simulink model "needle3"  (R2015a)
settings: Solver=ode45  StartTime=0.0  StopTime=10  FixedStep=0.01  RelTol=1e-3
settings Model: Creator=LAB425  LastModifiedBy=LAB425

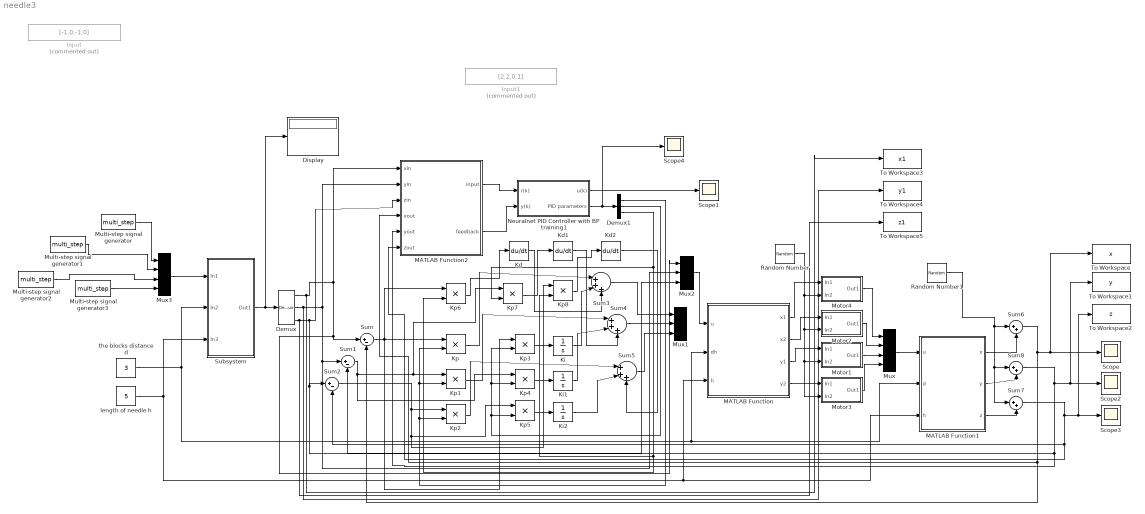
== system needle3 ==
  Demux : Demux  Outputs=3
  Demux1 : Demux  Outputs=3
  Display : Display
  Input : Constant  Commented=on  Value=[-1,0,-1,0]
  Input1 : Constant  Commented=on  Value=[2,2,0,1]
  Kd : Derivative
  Kd1 : Derivative
  Kd2 : Derivative
  "Ki " : Integrator
  Ki1 : Integrator
  Ki2 : Integrator
  Kp{,1..8} (9 alike) : Product
  MATLAB Function : MATLAB Function  TreatAsAtomicUnit=on
  MATLAB Function1 : MATLAB Function  TreatAsAtomicUnit=on
  MATLAB Function2 : MATLAB Function  TreatAsAtomicUnit=on
  Motor1 : Subsystem
  Motor2 : Subsystem
  Motor3 : Subsystem
  Motor4 : Subsystem
  Multi-step signal generator : S-Function  FunctionName=multi_step  Parameters=tTime,yStep  mask{tTime=[0,5], yStep=[-2,-1]}
      mask prompts: tTime "Time instances"; yStep "Step Values"
      mask init:
      | xx=repmat(tTime,2,1); yy=repmat(yStep,2,1);
      | xx=[xx(:)' 2*tTime(end)-tTime(end-1)];
      | yy=[0, yy(:)'];
      mask Display: plot(xx,yy)
  Multi-step signal generator1 : S-Function  FunctionName=multi_step  Parameters=tTime,yStep  mask{tTime=[0,5], yStep=[0.5,0]}
      mask prompts: tTime "Time instances"; yStep "Step Values"
      mask init:
      | xx=repmat(tTime,2,1); yy=repmat(yStep,2,1);
      | xx=[xx(:)' 2*tTime(end)-tTime(end-1)];
      | yy=[0, yy(:)'];
      mask Display: plot(xx,yy)
  Multi-step signal generator2 : S-Function  FunctionName=multi_step  Parameters=tTime,yStep  mask{tTime=[0,5], yStep=[-2,0]}
      mask prompts: tTime "Time instances"; yStep "Step Values"
      mask init:
      | xx=repmat(tTime,2,1); yy=repmat(yStep,2,1);
      | xx=[xx(:)' 2*tTime(end)-tTime(end-1)];
      | yy=[0, yy(:)'];
      mask Display: plot(xx,yy)
  Multi-step signal generator3 : S-Function  FunctionName=multi_step  Parameters=tTime,yStep  mask{tTime=[0,5], yStep=[1,0]}
      mask prompts: tTime "Time instances"; yStep "Step Values"
      mask init:
      | xx=repmat(tTime,2,1); yy=repmat(yStep,2,1);
      | xx=[xx(:)' 2*tTime(end)-tTime(end-1)];
      | yy=[0, yy(:)'];
      mask Display: plot(xx,yy)
  Mux : Mux
  Mux1 : Mux  Inputs=3
  Mux2 : Mux  Inputs=3
  Mux3 : Mux
  Neuralnet PID Controller with BP training1 : Subsystem  mask{xite=0.3, alfa=0.04, n_hidden=5, U_m=10, T=0.001, kFunc1=log-sigmoid, kFunc2=log-simoid}
      mask prompts: xite "The value of  xite"; alfa "The value of alfa"; n_hidden "number of hidden layer nodes"; U_m "Actuator Limit U_m"; T "Sampling period"; kFunc1 "Hidden Layer Trans Function"; kFunc2 "Output layer trans function"
      mask TypeOptions kFunc1: sigmoid | log-sigmoid
      mask TypeOptions kFunc2: sigmoid | log-simoid
      mask Display: disp('BP PID Controller')
  Random Number : RandomNumber  Variance=0.0005  SampleTime=0.01
  Random Number1 : RandomNumber  Variance=0.0005  Seed=1  SampleTime=0.01
  Scope{,1..4} (5 alike) : Scope
      Scope2 settings: SaveName=ScopeData2
      Scope3 settings: SaveName=ScopeData3
      Scope4 settings: SaveName=ScopeData4
  Subsystem : Subsystem
  Sum : Sum  Inputs=|+-
  Sum1 : Sum  Inputs=|+-
  Sum2 : Sum  Inputs=|+-
  Sum3 : Sum  Inputs=|+++
  Sum4 : Sum  Inputs=|+++
  Sum5 : Sum  Inputs=|+++
  Sum6 : Sum  Inputs=|++
  Sum7 : Sum  Inputs=|++
  Sum8 : Sum  Inputs=|++
  To Workspace : ToWorkspace  VariableName=x  SaveFormat=Timeseries  SampleTime=-1
  To Workspace1 : ToWorkspace  VariableName=y  SaveFormat=Timeseries  SampleTime=-1
  To Workspace2 : ToWorkspace  VariableName=z  SaveFormat=Timeseries  SampleTime=-1
  To Workspace3 : ToWorkspace  VariableName=x1  SaveFormat=Timeseries  SampleTime=-1
  To Workspace4 : ToWorkspace  VariableName=y1  SaveFormat=Timeseries  SampleTime=-1
  To Workspace5 : ToWorkspace  VariableName=z1  SaveFormat=Timeseries  SampleTime=-1
  length of needle h : Constant  Value=5
  the blocks distance d : Constant  Value=3
  wires:
  length of needle h/1 -> MATLAB Function/3(h), MATLAB Function1/3(h), Subsystem/3(In3)
  the blocks distance d/1 -> Subsystem/2(In2), MATLAB Function/2(dh), MATLAB Function1/2(d)
  Mux/1 -> MATLAB Function1/1(u)
  Motor3/1(Out1) -> Mux/4
  Mux3/1 -> Subsystem/1(In1)
  Subsystem/1(Out1) -> Display/1, Demux/1
  Random Number/1 -> Motor4/2(In2), Motor2/2(In2), Motor1/2(In2), Motor3/2(In2)
  MATLAB Function/4(y2) -> Motor3/1(In1)
  MATLAB Function/1(x1) -> Motor4/1(In1)
  MATLAB Function/2(x2) -> Motor2/1(In1)
  MATLAB Function/3(y1) -> Motor1/1(In1)
  Motor4/1(Out1) -> Mux/1
  Motor2/1(Out1) -> Mux/2
  Motor1/1(Out1) -> Mux/3
  Demux/2 -> To Workspace4/1, MATLAB Function2/2(yin), Mux2/2, Sum1/1
  Demux/3 -> To Workspace5/1, Mux2/3, Sum2/1, MATLAB Function2/3(zin)
  MATLAB Function2/2(feedback) -> Neuralnet PID Controller with BP training1/2(y(k))
  Neuralnet PID Controller with BP training1/2(PID parameters) -> Scope4/1, Demux1/1
  Sum/1 -> Kp6/1, Kp3/1, Kp/1
  Demux1/1 -> Kp/2, Kp1/2, Kp2/2
  Sum1/1 -> Kp7/1, Kp1/1, Kp4/1
  Sum2/1 -> Kp8/1, Kp5/1, Kp2/1
  Demux1/2 -> Kp3/2, Kp4/2, Kp5/2
  Kp3/1 -> "Ki "/1
  "Ki "/1 -> Sum3/2
  Kp/1 -> Sum3/1
  Kp4/1 -> Ki1/1
  Kp5/1 -> Ki2/1
  Kp1/1 -> Sum4/1
  Ki1/1 -> Sum4/2
  Sum3/1 -> Mux1/1
  Sum4/1 -> Mux1/2
  Sum5/1 -> Mux1/3
  Ki2/1 -> Sum5/2
  Kp2/1 -> Sum5/1
  Demux1/3 -> Kp8/2, Kp6/2, Kp7/2
  Kp6/1 -> Kd/1
  Kd/1 -> Sum3/3
  Kp7/1 -> Kd1/1
  Kd1/1 -> Sum4/3
  Kp8/1 -> Kd2/1
  Kd2/1 -> Sum5/3
  MATLAB Function2/1(input) -> Neuralnet PID Controller with BP training1/1(r(k))
  Demux/1 -> To Workspace3/1, MATLAB Function2/1(xin), Sum/1, Mux2/1
  Mux2/1 -> MATLAB Function/1(u)
  Neuralnet PID Controller with BP training1/1(u(k)) -> Scope1/1
  Random Number1/1 -> Sum7/1, Sum8/1, Sum6/1
  MATLAB Function1/1(x) -> Sum6/2
  Sum8/1 -> MATLAB Function2/5(yout), Sum1/2, To Workspace1/1, Scope2/1
  Sum7/1 -> MATLAB Function2/6(zout), Sum2/2, Scope3/1, To Workspace2/1
  MATLAB Function1/2(y) -> Sum8/2
  MATLAB Function1/3(z) -> Sum7/2
  Sum6/1 -> MATLAB Function2/4(xout), Sum/2, To Workspace/1, Scope/1
  Multi-step signal generator/1 -> Mux3/1
  Multi-step signal generator1/1 -> Mux3/2
  Multi-step signal generator2/1 -> Mux3/3
  Multi-step signal generator3/1 -> Mux3/4

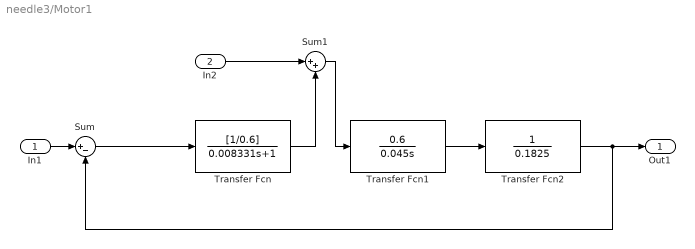
== system needle3/Motor1 ==
  In1 : Inport
  In2 : Inport  Port=2
  Sum : Sum  Inputs=|+-
  Sum1 : Sum  Inputs=|++
  Transfer Fcn : TransferFcn  Numerator=[1/0.6]  Denominator=[0.008331 1]
  Transfer Fcn1 : TransferFcn  Numerator=[0.6]  Denominator=[0.045 0]
  Transfer Fcn2 : TransferFcn  Denominator=[0.1825]
  Out1 : Outport
  wires:
  Transfer Fcn2/1 -> Sum/2, Out1/1
  Transfer Fcn1/1 -> Transfer Fcn2/1
  Sum1/1 -> Transfer Fcn1/1
  In2/1 -> Sum1/1
  Transfer Fcn/1 -> Sum1/2
  Sum/1 -> Transfer Fcn/1
  In1/1 -> Sum/1

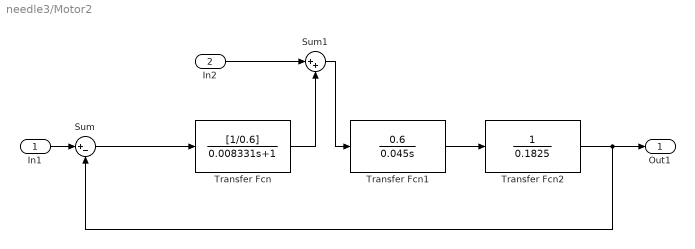
== system needle3/Motor2 ==
  In1 : Inport
  In2 : Inport  Port=2
  Sum : Sum  Inputs=|+-
  Sum1 : Sum  Inputs=|++
  Transfer Fcn : TransferFcn  Numerator=[1/0.6]  Denominator=[0.008331 1]
  Transfer Fcn1 : TransferFcn  Numerator=[0.6]  Denominator=[0.045 0]
  Transfer Fcn2 : TransferFcn  Denominator=[0.1825]
  Out1 : Outport
  wires:
  Transfer Fcn2/1 -> Sum/2, Out1/1
  Transfer Fcn1/1 -> Transfer Fcn2/1
  Sum1/1 -> Transfer Fcn1/1
  In2/1 -> Sum1/1
  Transfer Fcn/1 -> Sum1/2
  Sum/1 -> Transfer Fcn/1
  In1/1 -> Sum/1

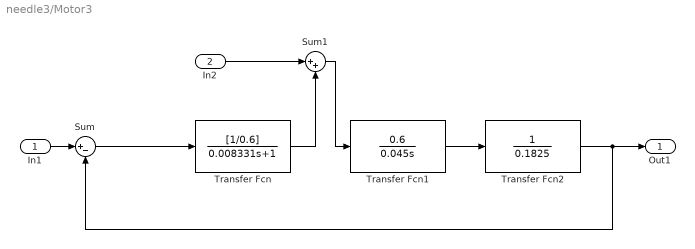
== system needle3/Motor3 ==
  In1 : Inport
  In2 : Inport  Port=2
  Sum : Sum  Inputs=|+-
  Sum1 : Sum  Inputs=|++
  Transfer Fcn : TransferFcn  Numerator=[1/0.6]  Denominator=[0.008331 1]
  Transfer Fcn1 : TransferFcn  Numerator=[0.6]  Denominator=[0.045 0]
  Transfer Fcn2 : TransferFcn  Denominator=[0.1825]
  Out1 : Outport
  wires:
  Transfer Fcn2/1 -> Sum/2, Out1/1
  Transfer Fcn1/1 -> Transfer Fcn2/1
  Sum1/1 -> Transfer Fcn1/1
  In2/1 -> Sum1/1
  Transfer Fcn/1 -> Sum1/2
  Sum/1 -> Transfer Fcn/1
  In1/1 -> Sum/1

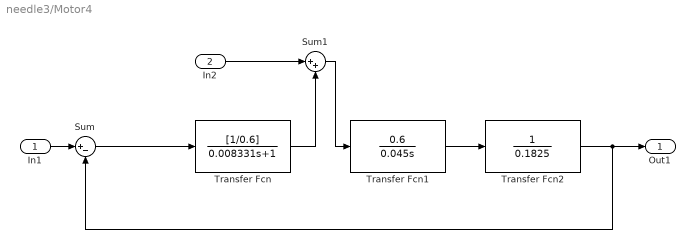
== system needle3/Motor4 ==
  In1 : Inport
  In2 : Inport  Port=2
  Sum : Sum  Inputs=|+-
  Sum1 : Sum  Inputs=|++
  Transfer Fcn : TransferFcn  Numerator=[1/0.6]  Denominator=[0.008331 1]
  Transfer Fcn1 : TransferFcn  Numerator=[0.6]  Denominator=[0.045 0]
  Transfer Fcn2 : TransferFcn  Denominator=[0.1825]
  Out1 : Outport
  wires:
  Transfer Fcn2/1 -> Sum/2, Out1/1
  Transfer Fcn1/1 -> Transfer Fcn2/1
  Sum1/1 -> Transfer Fcn1/1
  In2/1 -> Sum1/1
  Transfer Fcn/1 -> Sum1/2
  Sum/1 -> Transfer Fcn/1
  In1/1 -> Sum/1

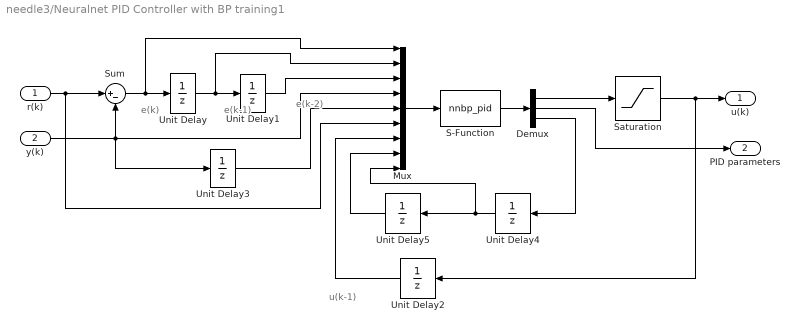
== system needle3/Neuralnet PID Controller with BP training1 ==
  note: e(k)
  note: e(k-1)
  note: e(k-2)
  note: u(k-1)
  r(k) : Inport
  y(k) : Inport  Port=2
  Demux : Demux  Outputs=[1,3,7*n_hidden]
  Mux : Mux  Inputs=9
  S-Function : S-Function  FunctionName=nnbp_pid  Parameters=T,n_hidden,xite,alfa,kFunc1,kFunc2
  Saturation : Saturate  UpperLimit=U_m  LowerLimit=-U_m
  Sum : Sum  Inputs=|+-  SaturateOnIntegerOverflow=on
  Unit Delay{,1..5} (6 alike) : UnitDelay  SampleTime=-1
  u(k) : Outport
  PID parameters : Outport  Port=2
  wires:
  Unit Delay5/1 -> Mux/8
  Demux/3 -> Unit Delay4/1
  Unit Delay4/1 -> Mux/9, Unit Delay5/1
  Unit Delay2/1 -> Mux/7
  Unit Delay1/1 -> Mux/3
  Unit Delay3/1 -> Mux/5
  Demux/2 -> PID parameters/1
  Demux/1 -> Saturation/1
  y(k)/1 -> Mux/4, Unit Delay3/1, Sum/2
  r(k)/1 -> Mux/6, Sum/1
  Saturation/1 -> Unit Delay2/1, u(k)/1
  S-Function/1 -> Demux/1
  Unit Delay/1 -> Mux/2, Unit Delay1/1
  Mux/1 -> S-Function/1
  Sum/1 -> Mux/1, Unit Delay/1

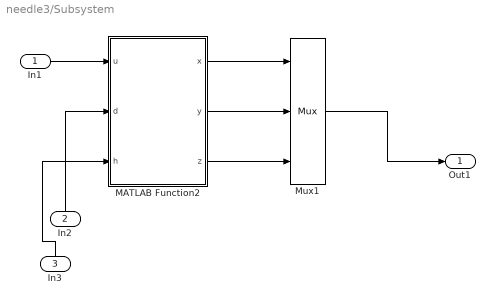
== system needle3/Subsystem ==
  In1 : Inport
  In2 : Inport  Port=2
  In3 : Inport  Port=3
  MATLAB Function2 : MATLAB Function  TreatAsAtomicUnit=on
  Mux1 : Mux  Inputs=3
  Out1 : Outport
  wires:
  MATLAB Function2/1(x) -> Mux1/1
  MATLAB Function2/2(y) -> Mux1/2
  Mux1/1 -> Out1/1
  MATLAB Function2/3(z) -> Mux1/3
  In1/1 -> MATLAB Function2/1(u)
  In2/1 -> MATLAB Function2/2(d)
  In3/1 -> MATLAB Function2/3(h)

== matlab function needle3/MATLAB Function1 ==
  data: x output; u input; y output; z output; d input; h input
function [x,y,z] = forward(u,d,h)
%#codegen

% y = u;
% mid = asin(u/5);
% 
% mid2 = 3 * tan(mid);
% 
% ymid = mid2 / 0.2;
% 
% y = pi * ymid;

x1 = u(1);x2 = u(2);y1 = u(3); y2 = u(4);

% T01=[1,0,0,0;0,cos(atan2((x1+x2),d)),-sin(atan2((x1+x2),d)),0;0,sin(atan2((x1+x2),d)),cos(atan2((x1+x2),d)),x1;0,0,0,1];
% T1m=[0,0,1,0;1,0,0,0,;0,1,0,0;0,0,0,1];
% Tmm1=[0,1,0,0;-1,0,0,0;0,0,1,0;0,0,0,1];
% Tm12=[1,0,0,0;0,cos(atan2((y1+y2),d))];
forwardx = sign(x1);forwardy = sign(y1);

X = abs(x1) + abs(x2);
Y = abs(y1) + abs(y2);
L = sqrt(X^2+Y^2);
theta = atan2(L,d);
H = h * sin(theta);
z = -h * cos(theta);
beta = atan2(Y,X);
y = -forwardy * (H * sin(beta) + abs(y2));
x = -forwardx * (H * cos(beta) + abs(x2));

== matlab function needle3/MATLAB Function ==
  data: u input; x1 output; dh input; h input; x2 output; y1 output; y2 output
function [x1,x2,y1,y2] = inv(u,dh,h)
%#codegen
% u = 2.5
% y = u;
limit = 2.774;
X=u(1);Y=u(2);Z=u(3);
forwardx = sign(X);forwardy=sign(Y);

if (-limit<= X && X <= limit) && (-limit<= Y && Y <= limit)
    X=abs(X);Y=abs(Y);
    beta = atan2(Y,X);
    H=sqrt(X^2+Y^2);
    theta=asin(H/h);
    D=dh*tan(theta);
    y1 = -forwardy * D * sin(beta);
    x1 = -forwardx * D * cos(beta);
    x2 = 0;
    y2 = 0;
else
    y1 = -forwardy * 2;x1 = -forwardx * 2;
    a = x1; 
    b = y1;
    d = Y; 
    c = X;
    B = h^2 - Z^2;
    D = real((dh * tan(acos(complex(abs(Z)/h)))))^2;
    E = (B - D - c^2 + a^2 - d^2 + b^2) / 2 ;
    F = a - c;
    G = b - d;
   
    EA = (F^2 + G^2)/G^2;
    EB = (2*G*d*F - 2*G^2*c - 2*E*F)/G^2;
    EC = (G^2*c^2 + G^2*d^2 - 2*G*d*E + E^2 - B*G^2)/G^2;
%     if (EB^2 - 4*EA*EC) < 0
%          y1 = -forwardy * 2;x1 = -forwardx * 2;
%          y2 = forwardy * 2;x2 = forwardx * 2;
    if sign((-EB + real(sqrt(complex(EB^2 - 4*EA*EC)))) / (2*EA)) == sign(forwardx)
        x2 = (-EB + real(sqrt(complex(EB^2 - 4*EA*EC)))) / (2*EA);
        y2 = (E - F*x2) / G;
    else
        x2 = (-EB - real(sqrt(complex(EB^2 - 4*EA*EC)))) / (2*EA);
        y2 = (E - F*x2) / G;
    end
end
%     X = abs(x1) + abs(x2);
%     Y = abs(y1) + abs(y2);
%     L = sqrt(X^2+Y^2);
%     theta = atan2(L,d);
%     H = h * sin(theta);
%     z = -h * cos(theta);
%     beta = atan2(Y,X);
%     y = -forwardy * (H * sin(beta) + abs(y2));
%     x = -forwardx * (H * cos(beta) + abs(x2));



% %     E = B - D - x^2 + x1^2 - y^2 + y1^2;
% %     F = 2*y1 + 2*y;
% %     G = 2*x1 + 2*x;
% %     A = F^2 + G^2;
% %     BB = 2*F*y1*G - 2*F^2*x1 - 2*E*G;
% %     C = F^2*x1^2 + F*y1^2 - 2*F*y1*E + E^2 - D*F^2;
% %     if (BB^2 - 4*A*C) < 0
% %         y1 = -forwardy * 2;x1 = -forwardx * 2;
% %         y2 = forwardy * 2;x2 = forwardx * 2;
% %     elseif (sign((-BB-sqrt(BB^2-4*A*C))/2*A) == sign(forwardx)) && ((-BB-sqrt(BB^2-4*A*C))/2*A <= 2) && ((-B-sqrt(B^2-4*A*C))/2*A >= -2)
% %         y1 = -forwardy * 2;x1 = -forwardx * 2;
% %         x2 = (-BB-sqrt(BB^2-4*A*C))/2*A;
% %         y2 = (E - G*x2)/F;
% %     else
% %         y1 = -forwardy * 2;x1 = -forwardx * 2;
% %         x2 = (-BB+sqrt(BB^2-4*A*C))/2*A;
% %         y2 = (E - G*x2)/F;
% %     end
%     A = (D-B+d^2+c^2-a^2-b^2)/2;
%     AA=(b-c)^2+(d-a)^2;
%     BB=2*A*(b-c)-2*b*(d-a)^2-2*a*(A+(b-c))*(d-a);
%     CC=A^2-(D-a^2-b^2)*(d-a)^2
% %     if (B^2 - 4*A*C) < 0
% %         y1 = -forwardy * 2;x1 = -forwardx * 2;
% %         y2 = forwardy * 2;x2 = forwardx * 2;
% %     elseif (sign((-B-sqrt(B^2-4*A*C))/2*A) == sign(forwardx)) && ((-B-sqrt(B^2-4*A*C))/2*A <= 2) && ((-B-sqrt(B^2-4*A*C))/2*A >= -2)
% %         y1 = -forwardy * 2;x1 = -forwardx * 2;
% %         x2 = (-B-sqrt(B^2-4*A*C))/2*A;
% %         y2 = 0;
% %     else
% %         y1 = -forwardy * 2;x1 = -forwardx * 2;
% %         x2 = (-B+sqrt(B^2-4*A*C))/2*A;
% %         y2 = 0;
% %     end
%      y1 = -forwardy * 2;x1 = -forwardx * 2;
%      x2 = (-BB + sqrt(BB^2 - 4 * AA * CC)) / 2 * AA;
%      y2=0;
end

== matlab function needle3/Subsystem/MATLAB Function2 ==
  data: x output; u input; y output; z output; d input; h input
function [x,y,z] = forward(u,d,h)
%#codegen

% y = u;
% mid = asin(u/5);
% 
% mid2 = 3 * tan(mid);
% 
% ymid = mid2 / 0.2;
% 
% y = pi * ymid;

x1 = u(1);x2 = u(2);y1 = u(3); y2 = u(4);

% T01=[1,0,0,0;0,cos(atan2((x1+x2),d)),-sin(atan2((x1+x2),d)),0;0,sin(atan2((x1+x2),d)),cos(atan2((x1+x2),d)),x1;0,0,0,1];
% T1m=[0,0,1,0;1,0,0,0,;0,1,0,0;0,0,0,1];
% Tmm1=[0,1,0,0;-1,0,0,0;0,0,1,0;0,0,0,1];
% Tm12=[1,0,0,0;0,cos(atan2((y1+y2),d))];
forwardx = sign(x1);forwardy = sign(y1);

X = abs(x1) + abs(x2);
Y = abs(y1) + abs(y2);
L = sqrt(X^2+Y^2);
theta = atan2(L,d);
H = h * sin(theta);
z = -h * cos(theta);
beta = atan2(Y,X);
y = -forwardy * (H * sin(beta) + abs(y2));
x = -forwardx * (H * cos(beta) + abs(x2));

== matlab function needle3/MATLAB Function2 ==
  data: xin input; input output; yin input; zin input; xout input; yout input; zout input; feedback output
function [input, feedback]  = distancexyz(xin, yin, zin, xout, yout, zout)
    
orign = sqrt(xin^2 + yin^2 + zin^2);
target = sqrt(xout^2 + yout^2 + zout^2);
input = orign;
feedback = target;
end
